simulink model "Online_Ordering_System_Functional_Architecture"  (R2025a)
settings: Solver=VariableStepAuto  StartTime=0.0  StopTime=10.0  RelTol=1e-3
model workspace (MAT data in the model file):
  Data : Simulink.Bus (value not decoded)
  ValueType : Simulink.ValueType (value not decoded)
(part 2 of 2)

== system Online_Ordering_System_Functional_Architecture/Process Order /Packaging Product ==
  Bus Element In1 : Inport  PortName=Packaging Products
  Bus Element Out1 : Outport  PortName=Update Information

== system Online_Ordering_System_Functional_Architecture/Process Order /Picking Up Product ==
  Bus Element In1 : Inport  PortName=Pick Up Product From Store
  Bus Element Out1 : Outport  PortName=Packaging Products

== system Online_Ordering_System_Functional_Architecture/Process Order /Validating Order ==
  Bus Element In1 : Inport  PortName=Process Order
  Bus Element Out1 : Outport  PortName=Checking Availibility

== system Online_Ordering_System_Functional_Architecture/Provide Customer Support/Collect Feedback ==

== system Online_Ordering_System_Functional_Architecture/Provide Customer Support/Live Customer Support ==

== system Online_Ordering_System_Functional_Architecture/Provide Customer Support/Send Discount Notification ==

== system Online_Ordering_System_Functional_Architecture/Provide Delivery Information/Display Delivery Information ==
  Bus Element In2 : Inport  PortName=Update Information
  Bus Element In1 : Inport  Port=2  PortName=Enter GPS Function
  Bus Element Out1 : Outport  PortName=Tracking Process

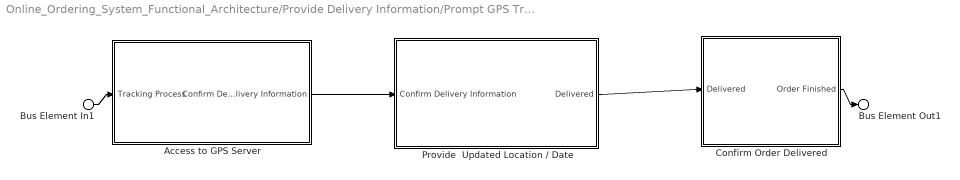
== system Online_Ordering_System_Functional_Architecture/Provide Delivery Information/Prompt GPS Tracking Function ==
  Bus Element In1 : Inport  PortName=Tracking Process
  Access to GPS Server : Subsystem
      settings: PortSchema="{\"entries\":[{\"content\":{\"headerSize\":26,\"margin\":15,\"minimumSpacing\":25,\"sides\":[{\"content\":{\"connectorIds\":[\"In1\"]},\"type\":\"ConnectorPlacement.EquallySpacedRectSide\",\"uuid\":\"9dfe17d1-9859-432c-bd2b-5498ec3a7f8d\"},{\"content\":{\"connectorIds\":[\"Out1\"],\"side\":\"RIGHT\"},\"type\":\"ConnectorPlacement.EquallySpacedRectSide\",\"uuid\":\"aa16792c-a675-4757-a131-98aa7729691b\"},{\"content\":{\"side\":\"TOP\"},\"type\":\"ConnectorPlacement.EquallySpacedRectSide\",\"uuid\":\"34f47498-03a7-4052-acac-71bdf4bb8cdc\"}]},\"type\":\"ConnectorPlacement.EquallySpacedConnector\",\"uuid\":\"11310cba-f92f-4ddc-beb4-2bbfc0816c51\"}],\"packageUris\":[\"http://schema.mathworks.com/mf0/Connector/R2020b\"],\"version\":\"1.0\"}"
  "Confirm Order Delivered  " : Subsystem
      settings: PortSchema="{\"entries\":[{\"content\":{\"headerSize\":26,\"margin\":15,\"minimumSpacing\":25,\"sides\":[{\"content\":{\"connectorIds\":[\"In1\"]},\"type\":\"ConnectorPlacement.EquallySpacedRectSide\",\"uuid\":\"427d1f3e-23ef-431e-830a-8ee80d1c0343\"},{\"content\":{\"connectorIds\":[\"Out1\"],\"side\":\"RIGHT\"},\"type\":\"ConnectorPlacement.EquallySpacedRectSide\",\"uuid\":\"a94733dc-dc80-40b7-a069-e69a5f529ec8\"},{\"content\":{\"side\":\"TOP\"},\"type\":\"ConnectorPlacement.EquallySpacedRectSide\",\"uuid\":\"aab6e856-7d0a-4bba-a547-38d5d593c589\"}]},\"type\":\"ConnectorPlacement.EquallySpacedConnector\",\"uuid\":\"17eb8191-1c5c-46d9-ae9e-c0a8464555a8\"}],\"packageUris\":[\"http://schema.mathworks.com/mf0/Connector/R2020b\"],\"version\":\"1.0\"}"
  Provide  Updated Location / Date : Subsystem
      settings: PortSchema="{\"entries\":[{\"content\":{\"headerSize\":26,\"margin\":15,\"minimumSpacing\":25,\"sides\":[{\"content\":{\"connectorIds\":[\"In1\"]},\"type\":\"ConnectorPlacement.EquallySpacedRectSide\",\"uuid\":\"427d1f3e-23ef-431e-830a-8ee80d1c0343\"},{\"content\":{\"connectorIds\":[\"Out1\"],\"side\":\"RIGHT\"},\"type\":\"ConnectorPlacement.EquallySpacedRectSide\",\"uuid\":\"a94733dc-dc80-40b7-a069-e69a5f529ec8\"},{\"content\":{\"side\":\"TOP\"},\"type\":\"ConnectorPlacement.EquallySpacedRectSide\",\"uuid\":\"aab6e856-7d0a-4bba-a547-38d5d593c589\"}]},\"type\":\"ConnectorPlacement.EquallySpacedConnector\",\"uuid\":\"17eb8191-1c5c-46d9-ae9e-c0a8464555a8\"}],\"packageUris\":[\"http://schema.mathworks.com/mf0/Connector/R2020b\"],\"version\":\"1.0\"}"
  Bus Element Out1 : Outport  PortName=Order Finished
  wires:
  Provide  Updated Location / Date/1(Delivered) -> "Confirm Order Delivered  "/1(Delivered)
  "Confirm Order Delivered  "/1(Order Finished) -> Bus Element Out1/1
  Bus Element In1/1 -> Access to GPS Server/1(Tracking Process)
  Access to GPS Server/1(Confirm Delivery Information) -> Provide  Updated Location / Date/1(Confirm Delivery Information)

== system Online_Ordering_System_Functional_Architecture/Set Up// Manage Account/Create New Customer Account ==
  Bus Element In1 : Inport  PortName=Enter System
  Bus Element Out1 : Outport  PortName=Access Customer Setting

== system Online_Ordering_System_Functional_Architecture/Set Up// Manage Account/Create New Merchant Account  ==
  Bus Element In1 : Inport  PortName=Enter System
  Bus Element Out1 : Outport  PortName=Access Merchant Setting

== system Online_Ordering_System_Functional_Architecture/Set Up// Manage Account/Enter // Edit Product  Menu ==
  Bus Element In1 : Inport  PortName=Access Product Management Page (Merchants)
  Bus Element Out1 : Outport  PortName=Modify Process

== system Online_Ordering_System_Functional_Architecture/Set Up// Manage Account/Enter // Edit Product  Price ==
  Bus Element In1 : Inport  PortName=Modify Process

== system Online_Ordering_System_Functional_Architecture/Set Up// Manage Account/Enter // Edit Product Description ==
  Bus Element In1 : Inport  PortName=Modify Process

== system Online_Ordering_System_Functional_Architecture/Set Up// Manage Account/Enter // Edit Product Images ==
  Bus Element In1 : Inport  PortName=Modify Process

== system Online_Ordering_System_Functional_Architecture/Set Up// Manage Account/Manage Customer Account Setting ==
  Bus Element In1 : Inport  PortName=Access Customer Setting

== system Online_Ordering_System_Functional_Architecture/Set Up// Manage Account/Manage Merchant Account Settings ==
  Bus Element In1 : Inport  PortName=Access Merchant Setting
  Bus Element Out2 : Outport  PortName=Access Product Management Page (Merchants)

== system Online_Ordering_System_Functional_Architecture/Payment Processing/Prompt Discounts & Rewords/Confirm Coupons // Rewords Selection ==
  Bus Element In1 : Inport  PortName=Select Discount
  Bus Element Out1 : Outport  PortName=Apply Discount

== system Online_Ordering_System_Functional_Architecture/Payment Processing/Prompt Discounts & Rewords/Display Counpons // Rewords Selection ==
  Bus Element In1 : Inport  PortName=Check Out With Discount
  Bus Element Out1 : Outport  PortName=Select Discount

== system Online_Ordering_System_Functional_Architecture/Provide Delivery Information/Prompt GPS Tracking Function/Access to GPS Server ==
  Bus Element In1 : Inport  PortName=Tracking Process
  Bus Element Out1 : Outport  PortName=Confirm Delivery Information

== system Online_Ordering_System_Functional_Architecture/Provide Delivery Information/Prompt GPS Tracking Function/Confirm Order Delivered   ==
  Bus Element In1 : Inport  PortName=Delivered
  Bus Element Out1 : Outport  PortName=Order Finished

== system Online_Ordering_System_Functional_Architecture/Provide Delivery Information/Prompt GPS Tracking Function/Provide  Updated Location // Date ==
  Bus Element In1 : Inport  PortName=Confirm Delivery Information
  Bus Element Out1 : Outport  PortName=Delivered
